simulink subsystem "reaction_wheel_model"  (R2025a)
settings: Solver=VariableStepAuto  StartTime=0.0  StopTime=10.0  RelTol=1e-3
undefined symbols (not defined in the file or in its folder): reaction_wheel_state_space_A, reaction_wheel_state_space_B, reaction_wheel_state_space_C, reaction_wheel_state_space_D, reaction_wheel_state_space_initial
settings Model: Creator=joshu  LastModifiedBy=arroy

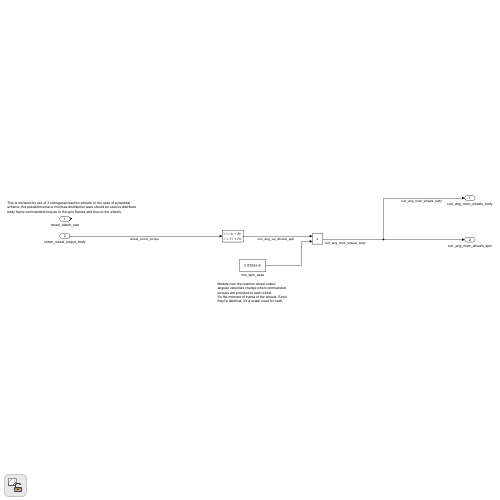
[thumbnail: Simulink's stored preview of the top-level diagram]
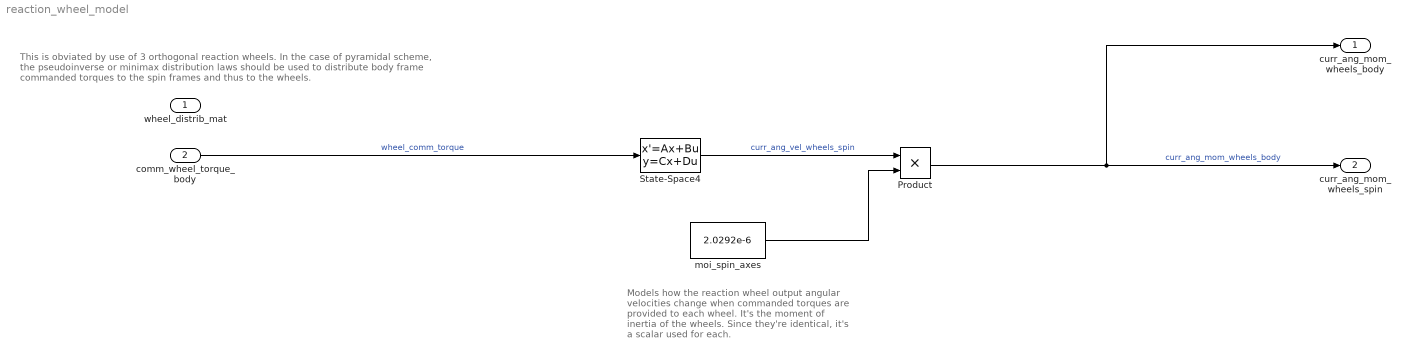
== system reaction_wheel_model ==
  note: This is obviated by use of 3 orthogonal reaction wheels. In the case of pyramidal
      | scheme, the pseudoinverse or minimax distribution laws should be used to distribute
      | body frame commanded torques to the spin frames and thus to the wheels.
  note: Models how the reaction wheel output angular velocities change when commanded torques are provided to each wheel.
      | It's the moment of inertia of the wheels. Since they're identical, it's a scalar used for each.
  wheel_distrib_mat : Inport
  comm_wheel_torque_body : Inport  Port=2
  Product : Product
  State-Space4 : StateSpace  A=reaction_wheel_state_space_A  B=reaction_wheel_state_space_B  C=reaction_wheel_state_space_C  D=reaction_wheel_state_space_D  InitialCondition=reaction_wheel_state_space_initial  ParameterTunability=Unconstrained
  moi_spin_axes : Constant  Value=2.0292e-6
  curr_ang_mom_wheels_body : Outport
  curr_ang_mom_wheels_spin : Outport  Port=2
  wires:
  moi_spin_axes/1 -> Product/2
  State-Space4/1 -> Product/1  "curr_ang_vel_wheels_spin"
  comm_wheel_torque_body/1 -> State-Space4/1  "wheel_comm_torque"
  Product/1 -> curr_ang_mom_wheels_spin/1, curr_ang_mom_wheels_body/1  "curr_ang_mom_wheels_body"
